simulink model "modele"  (R2021a)
settings: Solver=VariableStepAuto  StartTime=0.0  StopTime=10.0  RelTol=1e-3
settings Model: Creator=barto  LastModifiedBy=barto

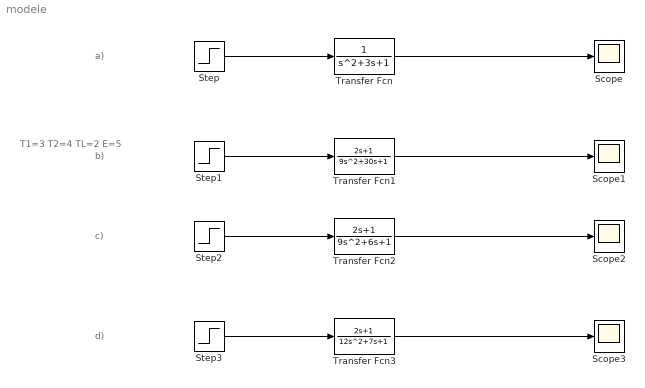
== system modele ==
  note: d)
  note: c)
  note: T1=3
      | T2=4
      | TL=2
      | E=5
  note: b)
  note: a)
  Scope{,1..3} (4 alike) : Scope
  Step{,1..3} (4 alike) : Step  Before=1  SampleTime=0
  Transfer Fcn : TransferFcn  Denominator=[1 3 1]
  Transfer Fcn1 : TransferFcn  Numerator=[2 1]  Denominator=[9 30 1]
  Transfer Fcn2 : TransferFcn  Numerator=[2 1]  Denominator=[9 6 1]
  Transfer Fcn3 : TransferFcn  Numerator=[2 1]  Denominator=[12 7 1]
  wires:
  Step/1 -> Transfer Fcn/1
  Transfer Fcn/1 -> Scope/1
  Step1/1 -> Transfer Fcn1/1
  Transfer Fcn1/1 -> Scope1/1
  Step2/1 -> Transfer Fcn2/1
  Transfer Fcn2/1 -> Scope2/1
  Step3/1 -> Transfer Fcn3/1
  Transfer Fcn3/1 -> Scope3/1
